simulink model "DatcomNew"  (R2017a)
settings: Solver=VariableStepAuto  StartTime=0.0  StopTime=10.0  RelTol=1e-3
undefined symbols (not defined in the file or in its folder): datcom, Newton, Raphson
libraries: aerolibutil x32, sharedutil x4, aerolibtransform2 x3, aerolibasang x3, aerolibadyn x1
(part 3 of 4)

== system DatcomNew/My Digital DATCOM v1.0.2/Deflection/Aerodynamic Forces and Moments/Force Transformation ==
  Vb : Inport
  Property-In-Stability (PIS) : Inport  Port=2
  Body2Stability : Subsystem
  "Incidence, Sideslip, & Airspeed" : Subsystem
      mask Display:
      | port_label('input',1,'V_b','texmode','on');
      | port_label('output',1,'\alpha','texmode','on');
      | port_label('output',2,'\beta','texmode','on');
      | port_label('output',3,'V','texmode','on');
  Product : Product  Multiplication=Matrix(*)  RndMeth=Zero
  Terminator : Terminator
  Terminator1 : Terminator
  Transpose : Math  Operator=transpose  SaturateOnIntegerOverflow=on
  Property-In-Body (PIB) : Outport
  wires:
  Product/1 -> Property-In-Body (PIB)/1
  Property-In-Stability (PIS)/1 -> Product/2
  "Incidence, Sideslip, & Airspeed"/1(Alpha) -> Body2Stability/1(alpha)
  Body2Stability/1(Ts/b) -> Transpose/1
  Transpose/1 -> Product/1  "Stability2Body"
  Vb/1 -> "Incidence, Sideslip, & Airspeed"/1(Vb)
  "Incidence, Sideslip, & Airspeed"/2(Beta) -> Terminator/1
  "Incidence, Sideslip, & Airspeed"/3(V) -> Terminator1/1

== system DatcomNew/My Digital DATCOM v1.0.2/Deflection/Aerodynamic Forces and Moments/Moment Transformation ==
  Vb : Inport
  Property-In-Stability (PIS) : Inport  Port=2
  Body2Stability : Subsystem
  "Incidence, Sideslip, & Airspeed" : Subsystem
      mask Display:
      | port_label('input',1,'V_b','texmode','on');
      | port_label('output',1,'\alpha','texmode','on');
      | port_label('output',2,'\beta','texmode','on');
      | port_label('output',3,'V','texmode','on');
  Product : Product  Multiplication=Matrix(*)  RndMeth=Zero
  Terminator : Terminator
  Terminator1 : Terminator
  Transpose : Math  Operator=transpose  SaturateOnIntegerOverflow=on
  Property-In-Body (PIB) : Outport
  wires:
  "Incidence, Sideslip, & Airspeed"/3(V) -> Terminator1/1
  "Incidence, Sideslip, & Airspeed"/2(Beta) -> Terminator/1
  Vb/1 -> "Incidence, Sideslip, & Airspeed"/1(Vb)
  Transpose/1 -> Product/1  "Stability2Body"
  Body2Stability/1(Ts/b) -> Transpose/1
  "Incidence, Sideslip, & Airspeed"/1(Alpha) -> Body2Stability/1(alpha)
  Property-In-Stability (PIS)/1 -> Product/2
  Product/1 -> Property-In-Body (PIB)/1

== system DatcomNew/My Digital DATCOM v1.0.2/Deflection/Delta Coefficients/Aileron Deflaction ==
  bus : Inport
  Bus Selector : BusSelector  OutputSignals=idxa,fa,idxm,fm,idxh,fh,idxd_a,fd_a
  Bus Selector1 : BusSelector  OutputSignals=idxa,fa,idxm,fm,idxh,fh,idxd_a,fd_a
  Constant{1,4..6} (4 alike) : Constant  Value=0
  DCl : Interpolation_n-D  NumberOfTableDimensions=4  Table=permute(datcom.dcl_de,[1 2 3 4])  RemoveProtectionIndex=on
      settings: InputPortMap=u0,u1,u2,u3,u4,u5,u6,u7
  DCn : Interpolation_n-D  NumberOfTableDimensions=4  Table=permute(datcom.dcdi_de,[1 2 3 4])  RemoveProtectionIndex=on
      settings: InputPortMap=u0,u1,u2,u3,u4,u5,u6,u7
  Mux1 : Mux  Inputs=6
  delCoeff_a : Outport
  wires:
  Bus Selector/7 -> DCn/7  "<idxd_a>"
  Bus Selector/3 -> DCn/3  "<idxm>"
  Bus Selector1/7 -> DCl/7  "<idxd_a>"
  Bus Selector1/3 -> DCl/3  "<idxm>"
  DCl/1 -> Mux1/4  "Cl_a"
  DCn/1 -> Mux1/6  "Cn_a"
  Constant6/1 -> Mux1/1  "CD_a"
  Constant1/1 -> Mux1/2  "CY_a"
  Constant5/1 -> Mux1/3  "CL_e"
  Constant4/1 -> Mux1/5  "Cm_a"
  bus/1 -> Bus Selector/1, Bus Selector1/1
  Bus Selector1/4 -> DCl/4  "<fm>"
  Bus Selector1/6 -> DCl/6  "<fh>"
  Bus Selector1/8 -> DCl/8  "<fd_a>"
  Bus Selector1/2 -> DCl/2  "<fa>"
  Bus Selector1/5 -> DCl/5  "<idxh>"
  Bus Selector1/1 -> DCl/1  "<idxa>"
  Mux1/1 -> delCoeff_a/1
  Bus Selector/6 -> DCn/6  "<fh>"
  Bus Selector/8 -> DCn/8  "<fd_a>"
  Bus Selector/1 -> DCn/1  "<idxa>"
  Bus Selector/2 -> DCn/2  "<fa>"
  Bus Selector/5 -> DCn/5  "<idxh>"
  Bus Selector/4 -> DCn/4  "<fm>"

== system DatcomNew/My Digital DATCOM v1.0.2/Deflection/Delta Coefficients/Elevator Deflaction ==
  bus : Inport
  Bus Selector : BusSelector  OutputSignals=idxa,fa,idxm,fm,idxh,fh,idxd_e,fd_e
  Bus Selector1 : BusSelector  OutputSignals=idxa,fa,idxm,fm,idxh,fh,idxd_e,fd_e
  Bus Selector2 : BusSelector  OutputSignals=idxa,fa,idxm,fm,idxh,fh,idxd_e,fd_e
  Constant1 : Constant  Value=0
  Constant2 : Constant  Value=0
  Constant3 : Constant  Value=0
  DCDI : Interpolation_n-D  NumberOfTableDimensions=4  Table=permute(datcom.dcdi_de,[1 2 3 4])  RemoveProtectionIndex=on
      settings: InputPortMap=u0,u1,u2,u3,u4,u5,u6,u7
  DCL : Interpolation_n-D  NumberOfTableDimensions=4  Table=permute(datcom.dcl_de,[1 2 3 4])  RemoveProtectionIndex=on
      settings: InputPortMap=u0,u1,u2,u3,u4,u5,u6,u7
  DCm : Interpolation_n-D  NumberOfTableDimensions=4  Table=permute(datcom.dcm_de,[1 2 3 4])  RemoveProtectionIndex=on
      settings: InputPortMap=u0,u1,u2,u3,u4,u5,u6,u7
  Mux1 : Mux  Inputs=6
  delCoeff_e : Outport
  wires:
  Bus Selector2/3 -> DCm/3  "<idxm>"
  Bus Selector2/7 -> DCm/7  "<idxd_e>"
  Bus Selector1/7 -> DCL/7  "<idxd_e>"
  Bus Selector1/3 -> DCL/3  "<idxm>"
  Bus Selector/3 -> DCDI/3  "<idxm>"
  Bus Selector/7 -> DCDI/7  "<idxd_e>"
  Constant2/1 -> Mux1/4  "Cl_e"
  Constant3/1 -> Mux1/6  "Cn_e"
  DCDI/1 -> Mux1/1  "CD_e"
  Constant1/1 -> Mux1/2  "CY_e"
  DCL/1 -> Mux1/3  "CL_e"
  DCm/1 -> Mux1/5  "Cm_e"
  Bus Selector/4 -> DCDI/4  "<fm>"
  Bus Selector/5 -> DCDI/5  "<idxh>"
  Bus Selector/2 -> DCDI/2  "<fa>"
  Bus Selector/1 -> DCDI/1  "<idxa>"
  Bus Selector/8 -> DCDI/8  "<fd_e>"
  Bus Selector/6 -> DCDI/6  "<fh>"
  Mux1/1 -> delCoeff_e/1
  Bus Selector1/1 -> DCL/1  "<idxa>"
  Bus Selector1/5 -> DCL/5  "<idxh>"
  Bus Selector1/2 -> DCL/2  "<fa>"
  Bus Selector2/1 -> DCm/1  "<idxa>"
  Bus Selector2/8 -> DCm/8  "<fd_e>"
  Bus Selector2/5 -> DCm/5  "<idxh>"
  Bus Selector2/4 -> DCm/4  "<fm>"
  Bus Selector2/2 -> DCm/2  "<fa>"
  Bus Selector2/6 -> DCm/6  "<fh>"
  Bus Selector1/8 -> DCL/8  "<fd_e>"
  Bus Selector1/6 -> DCL/6  "<fh>"
  Bus Selector1/4 -> DCL/4  "<fm>"
  bus/1 -> Bus Selector/1, Bus Selector1/1, Bus Selector2/1

== system DatcomNew/My Digital DATCOM v1.0.2/Deflection/Delta Coefficients/Flap Deflaction ==
  bus : Inport
  Bus Selector : BusSelector  OutputSignals=idxa,fa,idxm,fm,idxh,fh,idxd_f,fd_f
  Bus Selector1 : BusSelector  OutputSignals=idxa,fa,idxm,fm,idxh,fh,idxd_f,fd_f
  Bus Selector4 : BusSelector  OutputSignals=idxa,fa,idxm,fm,idxh,fh,idxd_f,fd_f
  Constant1 : Constant  Value=0
  Constant2 : Constant  Value=0
  Constant3 : Constant  Value=0
  DCDI : Interpolation_n-D  NumberOfTableDimensions=4  Table=permute(datcom.dcdi_df,[1 2 3 4])  RemoveProtectionIndex=on
      settings: InputPortMap=u0,u1,u2,u3,u4,u5,u6,u7
  DCL : Interpolation_n-D  NumberOfTableDimensions=4  Table=permute(datcom.dcl_df,[1 2 3 4])  RemoveProtectionIndex=on
      settings: InputPortMap=u0,u1,u2,u3,u4,u5,u6,u7
  DCm : Interpolation_n-D  NumberOfTableDimensions=4  Table=permute(datcom.dcm_df,[1 2 3 4])  RemoveProtectionIndex=on
      settings: InputPortMap=u0,u1,u2,u3,u4,u5,u6,u7
  Mux1 : Mux  Inputs=6
  delCoeff_f : Outport
  wires:
  Bus Selector4/3 -> DCm/3  "<idxm>"
  Bus Selector4/7 -> DCm/7  "<idxd_f>"
  Bus Selector1/7 -> DCL/7  "<idxd_f>"
  Bus Selector1/3 -> DCL/3  "<idxm>"
  Bus Selector/7 -> DCDI/7  "<idxd_f>"
  Bus Selector/3 -> DCDI/3  "<idxm>"
  Constant2/1 -> Mux1/4  "Cl_f"
  Constant3/1 -> Mux1/6  "Cn_f"
  bus/1 -> Bus Selector1/1, Bus Selector4/1, Bus Selector/1
  Bus Selector1/4 -> DCL/4  "<fm>"
  Bus Selector1/6 -> DCL/6  "<fh>"
  DCDI/1 -> Mux1/1  "CD_f"
  Constant1/1 -> Mux1/2  "CY_f"
  DCL/1 -> Mux1/3  "CL_f"
  Bus Selector1/8 -> DCL/8  "<fd_f>"
  Bus Selector4/6 -> DCm/6  "<fh>"
  Bus Selector4/2 -> DCm/2  "<fa>"
  Bus Selector4/4 -> DCm/4  "<fm>"
  Bus Selector4/5 -> DCm/5  "<idxh>"
  Bus Selector4/8 -> DCm/8  "<fd_f>"
  Bus Selector4/1 -> DCm/1  "<idxa>"
  Bus Selector1/2 -> DCL/2  "<fa>"
  Bus Selector1/5 -> DCL/5  "<idxh>"
  Bus Selector1/1 -> DCL/1  "<idxa>"
  DCm/1 -> Mux1/5  "Cm_f"
  Mux1/1 -> delCoeff_f/1
  Bus Selector/6 -> DCDI/6  "<fh>"
  Bus Selector/8 -> DCDI/8  "<fd_f>"
  Bus Selector/1 -> DCDI/1  "<idxa>"
  Bus Selector/2 -> DCDI/2  "<fa>"
  Bus Selector/5 -> DCDI/5  "<idxh>"
  Bus Selector/4 -> DCDI/4  "<fm>"

== system DatcomNew/My Digital DATCOM v1.0.2/Dynamic Contribution/Aerodynamic Forces and Moments Stability Axis/CG-CP Transformation ==
  Vb : Inport
  Property-In-Stability (PIS) : Inport  Port=2
  Body2Stability : Subsystem
  "Incidence, Sideslip, & Airspeed" : Subsystem
      mask Display:
      | port_label('input',1,'V_b','texmode','on');
      | port_label('output',1,'\alpha','texmode','on');
      | port_label('output',2,'\beta','texmode','on');
      | port_label('output',3,'V','texmode','on');
  Product : Product  Multiplication=Matrix(*)  RndMeth=Zero
  Terminator : Terminator
  Terminator1 : Terminator
  Transpose : Math  Operator=transpose  SaturateOnIntegerOverflow=on
  Property-In-Body (PIB) : Outport
  wires:
  Product/1 -> Property-In-Body (PIB)/1
  Property-In-Stability (PIS)/1 -> Product/2
  "Incidence, Sideslip, & Airspeed"/1(Alpha) -> Body2Stability/1(alpha)
  Body2Stability/1(Ts/b) -> Transpose/1
  Transpose/1 -> Product/1  "Stability2Body"
  Vb/1 -> "Incidence, Sideslip, & Airspeed"/1(Vb)
  "Incidence, Sideslip, & Airspeed"/2(Beta) -> Terminator/1
  "Incidence, Sideslip, & Airspeed"/3(V) -> Terminator1/1

== system DatcomNew/My Digital DATCOM v1.0.2/Dynamic Contribution/Aerodynamic Forces and Moments Stability Axis/Force Transformation ==
  Vb : Inport
  Property-In-Stability (PIS) : Inport  Port=2
  Body2Stability : Subsystem
  "Incidence, Sideslip, & Airspeed" : Subsystem
      mask Display:
      | port_label('input',1,'V_b','texmode','on');
      | port_label('output',1,'\alpha','texmode','on');
      | port_label('output',2,'\beta','texmode','on');
      | port_label('output',3,'V','texmode','on');
  Product : Product  Multiplication=Matrix(*)  RndMeth=Zero
  Terminator : Terminator
  Terminator1 : Terminator
  Transpose : Math  Operator=transpose  SaturateOnIntegerOverflow=on
  Property-In-Body (PIB) : Outport
  wires:
  Product/1 -> Property-In-Body (PIB)/1
  Property-In-Stability (PIS)/1 -> Product/2
  "Incidence, Sideslip, & Airspeed"/1(Alpha) -> Body2Stability/1(alpha)
  Body2Stability/1(Ts/b) -> Transpose/1
  Transpose/1 -> Product/1  "Stability2Body"
  Vb/1 -> "Incidence, Sideslip, & Airspeed"/1(Vb)
  "Incidence, Sideslip, & Airspeed"/2(Beta) -> Terminator/1
  "Incidence, Sideslip, & Airspeed"/3(V) -> Terminator1/1

== system DatcomNew/My Digital DATCOM v1.0.2/Dynamic Contribution/Aerodynamic Forces and Moments Stability Axis/Moment Transformation ==
  Vb : Inport
  Property-In-Stability (PIS) : Inport  Port=2
  Body2Stability : Subsystem
  "Incidence, Sideslip, & Airspeed" : Subsystem
      mask Display:
      | port_label('input',1,'V_b','texmode','on');
      | port_label('output',1,'\alpha','texmode','on');
      | port_label('output',2,'\beta','texmode','on');
      | port_label('output',3,'V','texmode','on');
  Product : Product  Multiplication=Matrix(*)  RndMeth=Zero
  Terminator : Terminator
  Terminator1 : Terminator
  Transpose : Math  Operator=transpose  SaturateOnIntegerOverflow=on
  Property-In-Body (PIB) : Outport
  wires:
  "Incidence, Sideslip, & Airspeed"/3(V) -> Terminator1/1
  "Incidence, Sideslip, & Airspeed"/2(Beta) -> Terminator/1
  Vb/1 -> "Incidence, Sideslip, & Airspeed"/1(Vb)
  Transpose/1 -> Product/1  "Stability2Body"
  Body2Stability/1(Ts/b) -> Transpose/1
  "Incidence, Sideslip, & Airspeed"/1(Alpha) -> Body2Stability/1(alpha)
  Property-In-Stability (PIS)/1 -> Product/2
  Product/1 -> Property-In-Body (PIB)/1

== system DatcomNew/My Digital DATCOM v1.0.2/Static Contribution/Aerodynamic Forces and Moments/CG-CP Transformation ==
  Vb : Inport
  Property-In-Stability (PIS) : Inport  Port=2
  Body2Stability : Subsystem
  "Incidence, Sideslip, & Airspeed" : Subsystem
      mask Display:
      | port_label('input',1,'V_b','texmode','on');
      | port_label('output',1,'\alpha','texmode','on');
      | port_label('output',2,'\beta','texmode','on');
      | port_label('output',3,'V','texmode','on');
  Product : Product  Multiplication=Matrix(*)  RndMeth=Zero
  Terminator : Terminator
  Terminator1 : Terminator
  Transpose : Math  Operator=transpose  SaturateOnIntegerOverflow=on
  Property-In-Body (PIB) : Outport
  wires:
  Product/1 -> Property-In-Body (PIB)/1
  Property-In-Stability (PIS)/1 -> Product/2
  "Incidence, Sideslip, & Airspeed"/1(Alpha) -> Body2Stability/1(alpha)
  Body2Stability/1(Ts/b) -> Transpose/1
  Transpose/1 -> Product/1  "Stability2Body"
  Vb/1 -> "Incidence, Sideslip, & Airspeed"/1(Vb)
  "Incidence, Sideslip, & Airspeed"/2(Beta) -> Terminator/1
  "Incidence, Sideslip, & Airspeed"/3(V) -> Terminator1/1

== system DatcomNew/My Digital DATCOM v1.0.2/Static Contribution/Aerodynamic Forces and Moments/Force Transformation ==
  Vb : Inport
  Property-In-Stability (PIS) : Inport  Port=2
  Body2Stability : Subsystem
  "Incidence, Sideslip, & Airspeed" : Subsystem
      mask Display:
      | port_label('input',1,'V_b','texmode','on');
      | port_label('output',1,'\alpha','texmode','on');
      | port_label('output',2,'\beta','texmode','on');
      | port_label('output',3,'V','texmode','on');
  Product : Product  Multiplication=Matrix(*)  RndMeth=Zero
  Terminator : Terminator
  Terminator1 : Terminator
  Transpose : Math  Operator=transpose  SaturateOnIntegerOverflow=on
  Property-In-Body (PIB) : Outport
  wires:
  Product/1 -> Property-In-Body (PIB)/1
  Property-In-Stability (PIS)/1 -> Product/2
  "Incidence, Sideslip, & Airspeed"/1(Alpha) -> Body2Stability/1(alpha)
  Body2Stability/1(Ts/b) -> Transpose/1
  Transpose/1 -> Product/1  "Stability2Body"
  Vb/1 -> "Incidence, Sideslip, & Airspeed"/1(Vb)
  "Incidence, Sideslip, & Airspeed"/2(Beta) -> Terminator/1
  "Incidence, Sideslip, & Airspeed"/3(V) -> Terminator1/1

== system DatcomNew/My Digital DATCOM v1.0.2/Static Contribution/Aerodynamic Forces and Moments/Moment Transformation ==
  Vb : Inport
  Property-In-Stability (PIS) : Inport  Port=2
  Body2Stability : Subsystem
  "Incidence, Sideslip, & Airspeed" : Subsystem
      mask Display:
      | port_label('input',1,'V_b','texmode','on');
      | port_label('output',1,'\alpha','texmode','on');
      | port_label('output',2,'\beta','texmode','on');
      | port_label('output',3,'V','texmode','on');
  Product : Product  Multiplication=Matrix(*)  RndMeth=Zero
  Terminator : Terminator
  Terminator1 : Terminator
  Transpose : Math  Operator=transpose  SaturateOnIntegerOverflow=on
  Property-In-Body (PIB) : Outport
  wires:
  "Incidence, Sideslip, & Airspeed"/3(V) -> Terminator1/1
  "Incidence, Sideslip, & Airspeed"/2(Beta) -> Terminator/1
  Vb/1 -> "Incidence, Sideslip, & Airspeed"/1(Vb)
  Transpose/1 -> Product/1  "Stability2Body"
  Body2Stability/1(Ts/b) -> Transpose/1
  "Incidence, Sideslip, & Airspeed"/1(Alpha) -> Body2Stability/1(alpha)
  Property-In-Stability (PIS)/1 -> Product/2
  Product/1 -> Property-In-Body (PIB)/1

== system DatcomNew/My Digital DATCOM v1.0.3/Deflection/Aerodynamic Forces and Moments/CG-CP Transformation ==
  Vb : Inport
  Property-In-Stability (PIS) : Inport  Port=2
  Body2Stability : Subsystem
  "Incidence, Sideslip, & Airspeed" : Subsystem
      mask Display:
      | port_label('input',1,'V_b','texmode','on');
      | port_label('output',1,'\alpha','texmode','on');
      | port_label('output',2,'\beta','texmode','on');
      | port_label('output',3,'V','texmode','on');
  Product : Product  Multiplication=Matrix(*)  RndMeth=Zero
  Terminator : Terminator
  Terminator1 : Terminator
  Transpose : Math  Operator=transpose  SaturateOnIntegerOverflow=on
  Property-In-Body (PIB) : Outport
  wires:
  Product/1 -> Property-In-Body (PIB)/1
  Property-In-Stability (PIS)/1 -> Product/2
  "Incidence, Sideslip, & Airspeed"/1(Alpha) -> Body2Stability/1(alpha)
  Body2Stability/1(Ts/b) -> Transpose/1
  Transpose/1 -> Product/1  "Stability2Body"
  Vb/1 -> "Incidence, Sideslip, & Airspeed"/1(Vb)
  "Incidence, Sideslip, & Airspeed"/2(Beta) -> Terminator/1
  "Incidence, Sideslip, & Airspeed"/3(V) -> Terminator1/1

== system DatcomNew/My Digital DATCOM v1.0.3/Deflection/Aerodynamic Forces and Moments/Force Transformation ==
  Vb : Inport
  Property-In-Stability (PIS) : Inport  Port=2
  Body2Stability : Subsystem
  "Incidence, Sideslip, & Airspeed" : Subsystem
      mask Display:
      | port_label('input',1,'V_b','texmode','on');
      | port_label('output',1,'\alpha','texmode','on');
      | port_label('output',2,'\beta','texmode','on');
      | port_label('output',3,'V','texmode','on');
  Product : Product  Multiplication=Matrix(*)  RndMeth=Zero
  Terminator : Terminator
  Terminator1 : Terminator
  Transpose : Math  Operator=transpose  SaturateOnIntegerOverflow=on
  Property-In-Body (PIB) : Outport
  wires:
  Product/1 -> Property-In-Body (PIB)/1
  Property-In-Stability (PIS)/1 -> Product/2
  "Incidence, Sideslip, & Airspeed"/1(Alpha) -> Body2Stability/1(alpha)
  Body2Stability/1(Ts/b) -> Transpose/1
  Transpose/1 -> Product/1  "Stability2Body"
  Vb/1 -> "Incidence, Sideslip, & Airspeed"/1(Vb)
  "Incidence, Sideslip, & Airspeed"/2(Beta) -> Terminator/1
  "Incidence, Sideslip, & Airspeed"/3(V) -> Terminator1/1

== system DatcomNew/My Digital DATCOM v1.0.3/Deflection/Aerodynamic Forces and Moments/Moment Transformation ==
  Vb : Inport
  Property-In-Stability (PIS) : Inport  Port=2
  Body2Stability : Subsystem
  "Incidence, Sideslip, & Airspeed" : Subsystem
      mask Display:
      | port_label('input',1,'V_b','texmode','on');
      | port_label('output',1,'\alpha','texmode','on');
      | port_label('output',2,'\beta','texmode','on');
      | port_label('output',3,'V','texmode','on');
  Product : Product  Multiplication=Matrix(*)  RndMeth=Zero
  Terminator : Terminator
  Terminator1 : Terminator
  Transpose : Math  Operator=transpose  SaturateOnIntegerOverflow=on
  Property-In-Body (PIB) : Outport
  wires:
  "Incidence, Sideslip, & Airspeed"/3(V) -> Terminator1/1
  "Incidence, Sideslip, & Airspeed"/2(Beta) -> Terminator/1
  Vb/1 -> "Incidence, Sideslip, & Airspeed"/1(Vb)
  Transpose/1 -> Product/1  "Stability2Body"
  Body2Stability/1(Ts/b) -> Transpose/1
  "Incidence, Sideslip, & Airspeed"/1(Alpha) -> Body2Stability/1(alpha)
  Property-In-Stability (PIS)/1 -> Product/2
  Product/1 -> Property-In-Body (PIB)/1

== system DatcomNew/My Digital DATCOM v1.0.3/Deflection/Delta Coefficients/Aileron Deflaction ==
  bus : Inport
  Bus Selector : BusSelector  OutputSignals=idxa,fa,idxm,fm,idxh,fh,idxd_a,fd_a
  Bus Selector1 : BusSelector  OutputSignals=idxa,fa,idxm,fm,idxh,fh,idxd_a,fd_a
  Constant{1,4..6} (4 alike) : Constant  Value=0
  DCl : Interpolation_n-D  NumberOfTableDimensions=4  Table=permute(datcom.dcl_de,[1 2 3 4])  RemoveProtectionIndex=on
      settings: InputPortMap=u0,u1,u2,u3,u4,u5,u6,u7
  DCn : Interpolation_n-D  NumberOfTableDimensions=4  Table=permute(datcom.dcdi_de,[1 2 3 4])  RemoveProtectionIndex=on
      settings: InputPortMap=u0,u1,u2,u3,u4,u5,u6,u7
  Mux1 : Mux  Inputs=6
  delCoeff_a : Outport
  wires:
  Bus Selector/7 -> DCn/7  "<idxd_a>"
  Bus Selector/3 -> DCn/3  "<idxm>"
  Bus Selector1/7 -> DCl/7  "<idxd_a>"
  Bus Selector1/3 -> DCl/3  "<idxm>"
  DCl/1 -> Mux1/4  "Cl_a"
  DCn/1 -> Mux1/6  "Cn_a"
  Constant6/1 -> Mux1/1  "CD_a"
  Constant1/1 -> Mux1/2  "CY_a"
  Constant5/1 -> Mux1/3  "CL_e"
  Constant4/1 -> Mux1/5  "Cm_a"
  bus/1 -> Bus Selector/1, Bus Selector1/1
  Bus Selector1/4 -> DCl/4  "<fm>"
  Bus Selector1/6 -> DCl/6  "<fh>"
  Bus Selector1/8 -> DCl/8  "<fd_a>"
  Bus Selector1/2 -> DCl/2  "<fa>"
  Bus Selector1/5 -> DCl/5  "<idxh>"
  Bus Selector1/1 -> DCl/1  "<idxa>"
  Mux1/1 -> delCoeff_a/1
  Bus Selector/6 -> DCn/6  "<fh>"
  Bus Selector/8 -> DCn/8  "<fd_a>"
  Bus Selector/1 -> DCn/1  "<idxa>"
  Bus Selector/2 -> DCn/2  "<fa>"
  Bus Selector/5 -> DCn/5  "<idxh>"
  Bus Selector/4 -> DCn/4  "<fm>"

== system DatcomNew/My Digital DATCOM v1.0.3/Deflection/Delta Coefficients/Elevator Deflaction ==
  bus : Inport
  Bus Selector : BusSelector  OutputSignals=idxa,fa,idxm,fm,idxh,fh,idxd_e,fd_e
  Bus Selector1 : BusSelector  OutputSignals=idxa,fa,idxm,fm,idxh,fh,idxd_e,fd_e
  Bus Selector2 : BusSelector  OutputSignals=idxa,fa,idxm,fm,idxh,fh,idxd_e,fd_e
  Constant1 : Constant  Value=0
  Constant2 : Constant  Value=0
  Constant3 : Constant  Value=0
  DCDI : Interpolation_n-D  NumberOfTableDimensions=4  Table=permute(datcom.dcdi_de,[1 2 3 4])  RemoveProtectionIndex=on
      settings: InputPortMap=u0,u1,u2,u3,u4,u5,u6,u7
  DCL : Interpolation_n-D  NumberOfTableDimensions=4  Table=permute(datcom.dcl_de,[1 2 3 4])  RemoveProtectionIndex=on
      settings: InputPortMap=u0,u1,u2,u3,u4,u5,u6,u7
  DCm : Interpolation_n-D  NumberOfTableDimensions=4  Table=permute(datcom.dcm_de,[1 2 3 4])  RemoveProtectionIndex=on
      settings: InputPortMap=u0,u1,u2,u3,u4,u5,u6,u7
  Mux1 : Mux  Inputs=6
  delCoeff_e : Outport
  wires:
  Bus Selector2/3 -> DCm/3  "<idxm>"
  Bus Selector2/7 -> DCm/7  "<idxd_e>"
  Bus Selector1/7 -> DCL/7  "<idxd_e>"
  Bus Selector1/3 -> DCL/3  "<idxm>"
  Bus Selector/3 -> DCDI/3  "<idxm>"
  Bus Selector/7 -> DCDI/7  "<idxd_e>"
  Constant2/1 -> Mux1/4  "Cl_e"
  Constant3/1 -> Mux1/6  "Cn_e"
  DCDI/1 -> Mux1/1  "CD_e"
  Constant1/1 -> Mux1/2  "CY_e"
  DCL/1 -> Mux1/3  "CL_e"
  DCm/1 -> Mux1/5  "Cm_e"
  Bus Selector/4 -> DCDI/4  "<fm>"
  Bus Selector/5 -> DCDI/5  "<idxh>"
  Bus Selector/2 -> DCDI/2  "<fa>"
  Bus Selector/1 -> DCDI/1  "<idxa>"
  Bus Selector/8 -> DCDI/8  "<fd_e>"
  Bus Selector/6 -> DCDI/6  "<fh>"
  Mux1/1 -> delCoeff_e/1
  Bus Selector1/1 -> DCL/1  "<idxa>"
  Bus Selector1/5 -> DCL/5  "<idxh>"
  Bus Selector1/2 -> DCL/2  "<fa>"
  Bus Selector2/1 -> DCm/1  "<idxa>"
  Bus Selector2/8 -> DCm/8  "<fd_e>"
  Bus Selector2/5 -> DCm/5  "<idxh>"
  Bus Selector2/4 -> DCm/4  "<fm>"
  Bus Selector2/2 -> DCm/2  "<fa>"
  Bus Selector2/6 -> DCm/6  "<fh>"
  Bus Selector1/8 -> DCL/8  "<fd_e>"
  Bus Selector1/6 -> DCL/6  "<fh>"
  Bus Selector1/4 -> DCL/4  "<fm>"
  bus/1 -> Bus Selector/1, Bus Selector1/1, Bus Selector2/1

== system DatcomNew/My Digital DATCOM v1.0.3/Deflection/Delta Coefficients/Flap Deflaction ==
  bus : Inport
  Bus Selector : BusSelector  OutputSignals=idxa,fa,idxm,fm,idxh,fh,idxd_f,fd_f
  Bus Selector1 : BusSelector  OutputSignals=idxa,fa,idxm,fm,idxh,fh,idxd_f,fd_f
  Bus Selector4 : BusSelector  OutputSignals=idxa,fa,idxm,fm,idxh,fh,idxd_f,fd_f
  Constant1 : Constant  Value=0
  Constant2 : Constant  Value=0
  Constant3 : Constant  Value=0
  DCDI : Interpolation_n-D  NumberOfTableDimensions=4  Table=permute(datcom.dcdi_df,[1 2 3 4])  RemoveProtectionIndex=on
      settings: InputPortMap=u0,u1,u2,u3,u4,u5,u6,u7
  DCL : Interpolation_n-D  NumberOfTableDimensions=4  Table=permute(datcom.dcl_df,[1 2 3 4])  RemoveProtectionIndex=on
      settings: InputPortMap=u0,u1,u2,u3,u4,u5,u6,u7
  DCm : Interpolation_n-D  NumberOfTableDimensions=4  Table=permute(datcom.dcm_df,[1 2 3 4])  RemoveProtectionIndex=on
      settings: InputPortMap=u0,u1,u2,u3,u4,u5,u6,u7
  Mux1 : Mux  Inputs=6
  delCoeff_f : Outport
  wires:
  Bus Selector4/3 -> DCm/3  "<idxm>"
  Bus Selector4/7 -> DCm/7  "<idxd_f>"
  Bus Selector1/7 -> DCL/7  "<idxd_f>"
  Bus Selector1/3 -> DCL/3  "<idxm>"
  Bus Selector/7 -> DCDI/7  "<idxd_f>"
  Bus Selector/3 -> DCDI/3  "<idxm>"
  Constant2/1 -> Mux1/4  "Cl_f"
  Constant3/1 -> Mux1/6  "Cn_f"
  bus/1 -> Bus Selector1/1, Bus Selector4/1, Bus Selector/1
  Bus Selector1/4 -> DCL/4  "<fm>"
  Bus Selector1/6 -> DCL/6  "<fh>"
  DCDI/1 -> Mux1/1  "CD_f"
  Constant1/1 -> Mux1/2  "CY_f"
  DCL/1 -> Mux1/3  "CL_f"
  Bus Selector1/8 -> DCL/8  "<fd_f>"
  Bus Selector4/6 -> DCm/6  "<fh>"
  Bus Selector4/2 -> DCm/2  "<fa>"
  Bus Selector4/4 -> DCm/4  "<fm>"
  Bus Selector4/5 -> DCm/5  "<idxh>"
  Bus Selector4/8 -> DCm/8  "<fd_f>"
  Bus Selector4/1 -> DCm/1  "<idxa>"
  Bus Selector1/2 -> DCL/2  "<fa>"
  Bus Selector1/5 -> DCL/5  "<idxh>"
  Bus Selector1/1 -> DCL/1  "<idxa>"
  DCm/1 -> Mux1/5  "Cm_f"
  Mux1/1 -> delCoeff_f/1
  Bus Selector/6 -> DCDI/6  "<fh>"
  Bus Selector/8 -> DCDI/8  "<fd_f>"
  Bus Selector/1 -> DCDI/1  "<idxa>"
  Bus Selector/2 -> DCDI/2  "<fa>"
  Bus Selector/5 -> DCDI/5  "<idxh>"
  Bus Selector/4 -> DCDI/4  "<fm>"

== system DatcomNew/My Digital DATCOM v1.0.3/Dynamic Contribution/Aerodynamic Forces and Moments Stability Axis/CG-CP Transformation ==
  Vb : Inport
  Property-In-Stability (PIS) : Inport  Port=2
  Body2Stability : Subsystem
  "Incidence, Sideslip, & Airspeed" : Subsystem
      mask Display:
      | port_label('input',1,'V_b','texmode','on');
      | port_label('output',1,'\alpha','texmode','on');
      | port_label('output',2,'\beta','texmode','on');
      | port_label('output',3,'V','texmode','on');
  Product : Product  Multiplication=Matrix(*)  RndMeth=Zero
  Terminator : Terminator
  Terminator1 : Terminator
  Transpose : Math  Operator=transpose  SaturateOnIntegerOverflow=on
  Property-In-Body (PIB) : Outport
  wires:
  Product/1 -> Property-In-Body (PIB)/1
  Property-In-Stability (PIS)/1 -> Product/2
  "Incidence, Sideslip, & Airspeed"/1(Alpha) -> Body2Stability/1(alpha)
  Body2Stability/1(Ts/b) -> Transpose/1
  Transpose/1 -> Product/1  "Stability2Body"
  Vb/1 -> "Incidence, Sideslip, & Airspeed"/1(Vb)
  "Incidence, Sideslip, & Airspeed"/2(Beta) -> Terminator/1
  "Incidence, Sideslip, & Airspeed"/3(V) -> Terminator1/1

== system DatcomNew/My Digital DATCOM v1.0.3/Dynamic Contribution/Aerodynamic Forces and Moments Stability Axis/Force Transformation ==
  Vb : Inport
  Property-In-Stability (PIS) : Inport  Port=2
  Body2Stability : Subsystem
  "Incidence, Sideslip, & Airspeed" : Subsystem
      mask Display:
      | port_label('input',1,'V_b','texmode','on');
      | port_label('output',1,'\alpha','texmode','on');
      | port_label('output',2,'\beta','texmode','on');
      | port_label('output',3,'V','texmode','on');
  Product : Product  Multiplication=Matrix(*)  RndMeth=Zero
  Terminator : Terminator
  Terminator1 : Terminator
  Transpose : Math  Operator=transpose  SaturateOnIntegerOverflow=on
  Property-In-Body (PIB) : Outport
  wires:
  Product/1 -> Property-In-Body (PIB)/1
  Property-In-Stability (PIS)/1 -> Product/2
  "Incidence, Sideslip, & Airspeed"/1(Alpha) -> Body2Stability/1(alpha)
  Body2Stability/1(Ts/b) -> Transpose/1
  Transpose/1 -> Product/1  "Stability2Body"
  Vb/1 -> "Incidence, Sideslip, & Airspeed"/1(Vb)
  "Incidence, Sideslip, & Airspeed"/2(Beta) -> Terminator/1
  "Incidence, Sideslip, & Airspeed"/3(V) -> Terminator1/1

== system DatcomNew/My Digital DATCOM v1.0.3/Dynamic Contribution/Aerodynamic Forces and Moments Stability Axis/Moment Transformation ==
  Vb : Inport
  Property-In-Stability (PIS) : Inport  Port=2
  Body2Stability : Subsystem
  "Incidence, Sideslip, & Airspeed" : Subsystem
      mask Display:
      | port_label('input',1,'V_b','texmode','on');
      | port_label('output',1,'\alpha','texmode','on');
      | port_label('output',2,'\beta','texmode','on');
      | port_label('output',3,'V','texmode','on');
  Product : Product  Multiplication=Matrix(*)  RndMeth=Zero
  Terminator : Terminator
  Terminator1 : Terminator
  Transpose : Math  Operator=transpose  SaturateOnIntegerOverflow=on
  Property-In-Body (PIB) : Outport
  wires:
  "Incidence, Sideslip, & Airspeed"/3(V) -> Terminator1/1
  "Incidence, Sideslip, & Airspeed"/2(Beta) -> Terminator/1
  Vb/1 -> "Incidence, Sideslip, & Airspeed"/1(Vb)
  Transpose/1 -> Product/1  "Stability2Body"
  Body2Stability/1(Ts/b) -> Transpose/1
  "Incidence, Sideslip, & Airspeed"/1(Alpha) -> Body2Stability/1(alpha)
  Property-In-Stability (PIS)/1 -> Product/2
  Product/1 -> Property-In-Body (PIB)/1

== system DatcomNew/My Digital DATCOM v1.0.3/Static Contribution/Aerodynamic Forces and Moments/CG-CP Transformation ==
  Vb : Inport
  Property-In-Stability (PIS) : Inport  Port=2
  Body2Stability : Subsystem
  "Incidence, Sideslip, & Airspeed" : Subsystem
      mask Display:
      | port_label('input',1,'V_b','texmode','on');
      | port_label('output',1,'\alpha','texmode','on');
      | port_label('output',2,'\beta','texmode','on');
      | port_label('output',3,'V','texmode','on');
  Product : Product  Multiplication=Matrix(*)  RndMeth=Zero
  Terminator : Terminator
  Terminator1 : Terminator
  Transpose : Math  Operator=transpose  SaturateOnIntegerOverflow=on
  Property-In-Body (PIB) : Outport
  wires:
  Product/1 -> Property-In-Body (PIB)/1
  Property-In-Stability (PIS)/1 -> Product/2
  "Incidence, Sideslip, & Airspeed"/1(Alpha) -> Body2Stability/1(alpha)
  Body2Stability/1(Ts/b) -> Transpose/1
  Transpose/1 -> Product/1  "Stability2Body"
  Vb/1 -> "Incidence, Sideslip, & Airspeed"/1(Vb)
  "Incidence, Sideslip, & Airspeed"/2(Beta) -> Terminator/1
  "Incidence, Sideslip, & Airspeed"/3(V) -> Terminator1/1

== system DatcomNew/My Digital DATCOM v1.0.3/Static Contribution/Aerodynamic Forces and Moments/Force Transformation ==
  Vb : Inport
  Property-In-Stability (PIS) : Inport  Port=2
  Body2Stability : Subsystem
  "Incidence, Sideslip, & Airspeed" : Subsystem
      mask Display:
      | port_label('input',1,'V_b','texmode','on');
      | port_label('output',1,'\alpha','texmode','on');
      | port_label('output',2,'\beta','texmode','on');
      | port_label('output',3,'V','texmode','on');
  Product : Product  Multiplication=Matrix(*)  RndMeth=Zero
  Terminator : Terminator
  Terminator1 : Terminator
  Transpose : Math  Operator=transpose  SaturateOnIntegerOverflow=on
  Property-In-Body (PIB) : Outport
  wires:
  Product/1 -> Property-In-Body (PIB)/1
  Property-In-Stability (PIS)/1 -> Product/2
  "Incidence, Sideslip, & Airspeed"/1(Alpha) -> Body2Stability/1(alpha)
  Body2Stability/1(Ts/b) -> Transpose/1
  Transpose/1 -> Product/1  "Stability2Body"
  Vb/1 -> "Incidence, Sideslip, & Airspeed"/1(Vb)
  "Incidence, Sideslip, & Airspeed"/2(Beta) -> Terminator/1
  "Incidence, Sideslip, & Airspeed"/3(V) -> Terminator1/1

== system DatcomNew/My Digital DATCOM v1.0.3/Static Contribution/Aerodynamic Forces and Moments/Moment Transformation ==
  Vb : Inport
  Property-In-Stability (PIS) : Inport  Port=2
  Body2Stability : Subsystem
  "Incidence, Sideslip, & Airspeed" : Subsystem
      mask Display:
      | port_label('input',1,'V_b','texmode','on');
      | port_label('output',1,'\alpha','texmode','on');
      | port_label('output',2,'\beta','texmode','on');
      | port_label('output',3,'V','texmode','on');
  Product : Product  Multiplication=Matrix(*)  RndMeth=Zero
  Terminator : Terminator
  Terminator1 : Terminator
  Transpose : Math  Operator=transpose  SaturateOnIntegerOverflow=on
  Property-In-Body (PIB) : Outport
  wires:
  "Incidence, Sideslip, & Airspeed"/3(V) -> Terminator1/1
  "Incidence, Sideslip, & Airspeed"/2(Beta) -> Terminator/1
  Vb/1 -> "Incidence, Sideslip, & Airspeed"/1(Vb)
  Transpose/1 -> Product/1  "Stability2Body"
  Body2Stability/1(Ts/b) -> Transpose/1
  "Incidence, Sideslip, & Airspeed"/1(Alpha) -> Body2Stability/1(alpha)
  Property-In-Stability (PIS)/1 -> Product/2
  Product/1 -> Property-In-Body (PIB)/1

== system DatcomNew/My Digital DATCOM v1.0.1/Deflection/Aerodynamic Forces and Moments/CG-CP Transformation/Body2Stability ==
  alpha : Inport
  Constant{,1,3..4} (4 alike) : Constant  Value=0
  Constant2 : Constant
  Create 3x3 Matrix : aerolibutil/Create 3x3 Matrix
      settings: SourceProductName=Aerospace Blockset  SourceProductBaseCode=AE
  Trigonometric Function2 : Trigonometry  Operator=sincos
  Unary Minus : UnaryMinus
  Ts/b : Outport
  wires:
  Create 3x3 Matrix/1 -> Ts/b/1
  Constant/1 -> Create 3x3 Matrix/2
  Constant1/1 -> Create 3x3 Matrix/4
  Constant2/1 -> Create 3x3 Matrix/5
  Constant3/1 -> Create 3x3 Matrix/6
  Trigonometric Function2/1 -> Create 3x3 Matrix/3, Unary Minus/1
  Unary Minus/1 -> Create 3x3 Matrix/7
  Constant4/1 -> Create 3x3 Matrix/8
  Trigonometric Function2/2 -> Create 3x3 Matrix/1, Create 3x3 Matrix/9
  alpha/1 -> Trigonometric Function2/1

== system DatcomNew/My Digital DATCOM v1.0.1/Deflection/Aerodynamic Forces and Moments/CG-CP Transformation/Incidence, Sideslip, & Airspeed ==
  Vb : Inport  Unit=m/s
  Airspeed : Sqrt  AlgorithmType=Newton-Raphson  SaturateOnIntegerOverflow=on
  Dot Product : DotProduct  InputSameDT=on  OutDataTypeStr=Inherit: Inherit via internal rule
  Incidence : Trigonometry  Operator=atan2
  Product : Product  Inputs=*/  SaturateOnIntegerOverflow=on  OutDataTypeStr=Inherit: Same as first input
  Selector : Selector  InputPortWidth=3  IndexOptions=Index vector (dialog)  Indices=[2]  OutputSizes=1
  Selector1 : Selector  InputPortWidth=3  IndexOptions=Index vector (dialog)  Indices=[3]  OutputSizes=1
  Selector2 : Selector  InputPortWidth=3  IndexOptions=Index vector (dialog)  Indices=[1]  OutputSizes=1
  Sideslip : Trigonometry  Operator=asin
  Alpha : Outport  Unit=rad  InitialOutput=0
  Beta : Outport  Port=2  Unit=rad  InitialOutput=0
  V : Outport  Port=3  Unit=m/s  InitialOutput=0
  wires:
  Product/1 -> Sideslip/1
  Selector1/1 -> Incidence/1
  Selector2/1 -> Incidence/2
  Dot Product/1 -> Airspeed/1
  Airspeed/1 -> Product/2, V/1
  Incidence/1 -> Alpha/1
  Vb/1 -> Selector1/1, Selector2/1, Selector/1, Dot Product/1, Dot Product/2
  Sideslip/1 -> Beta/1
  Selector/1 -> Product/1

== system DatcomNew/My Digital DATCOM v1.0.1/Deflection/Aerodynamic Forces and Moments/Force Transformation/Body2Stability ==
  alpha : Inport
  Constant{,1,3..4} (4 alike) : Constant  Value=0
  Constant2 : Constant
  Create 3x3 Matrix : aerolibutil/Create 3x3 Matrix
      settings: SourceProductName=Aerospace Blockset  SourceProductBaseCode=AE
  Trigonometric Function2 : Trigonometry  Operator=sincos
  Unary Minus : UnaryMinus
  Ts/b : Outport
  wires:
  Create 3x3 Matrix/1 -> Ts/b/1
  Constant/1 -> Create 3x3 Matrix/2
  Constant1/1 -> Create 3x3 Matrix/4
  Constant2/1 -> Create 3x3 Matrix/5
  Constant3/1 -> Create 3x3 Matrix/6
  Trigonometric Function2/1 -> Create 3x3 Matrix/3, Unary Minus/1
  Unary Minus/1 -> Create 3x3 Matrix/7
  Constant4/1 -> Create 3x3 Matrix/8
  Trigonometric Function2/2 -> Create 3x3 Matrix/1, Create 3x3 Matrix/9
  alpha/1 -> Trigonometric Function2/1

== system DatcomNew/My Digital DATCOM v1.0.1/Deflection/Aerodynamic Forces and Moments/Force Transformation/Incidence, Sideslip, & Airspeed ==
  Vb : Inport  Unit=m/s
  Airspeed : Sqrt  AlgorithmType=Newton-Raphson  SaturateOnIntegerOverflow=on
  Dot Product : DotProduct  InputSameDT=on  OutDataTypeStr=Inherit: Inherit via internal rule
  Incidence : Trigonometry  Operator=atan2
  Product : Product  Inputs=*/  SaturateOnIntegerOverflow=on  OutDataTypeStr=Inherit: Same as first input
  Selector : Selector  InputPortWidth=3  IndexOptions=Index vector (dialog)  Indices=[2]  OutputSizes=1
  Selector1 : Selector  InputPortWidth=3  IndexOptions=Index vector (dialog)  Indices=[3]  OutputSizes=1
  Selector2 : Selector  InputPortWidth=3  IndexOptions=Index vector (dialog)  Indices=[1]  OutputSizes=1
  Sideslip : Trigonometry  Operator=asin
  Alpha : Outport  Unit=rad  InitialOutput=0
  Beta : Outport  Port=2  Unit=rad  InitialOutput=0
  V : Outport  Port=3  Unit=m/s  InitialOutput=0
  wires:
  Product/1 -> Sideslip/1
  Selector1/1 -> Incidence/1
  Selector2/1 -> Incidence/2
  Dot Product/1 -> Airspeed/1
  Airspeed/1 -> Product/2, V/1
  Incidence/1 -> Alpha/1
  Vb/1 -> Selector1/1, Selector2/1, Selector/1, Dot Product/1, Dot Product/2
  Sideslip/1 -> Beta/1
  Selector/1 -> Product/1

== system DatcomNew/My Digital DATCOM v1.0.1/Deflection/Aerodynamic Forces and Moments/Moment Transformation/Body2Stability ==
  alpha : Inport
  Constant{,1,3..4} (4 alike) : Constant  Value=0
  Constant2 : Constant
  Create 3x3 Matrix : aerolibutil/Create 3x3 Matrix
      settings: SourceProductName=Aerospace Blockset  SourceProductBaseCode=AE
  Trigonometric Function2 : Trigonometry  Operator=sincos
  Unary Minus : UnaryMinus
  Ts/b : Outport
  wires:
  alpha/1 -> Trigonometric Function2/1
  Trigonometric Function2/2 -> Create 3x3 Matrix/9, Create 3x3 Matrix/1
  Constant4/1 -> Create 3x3 Matrix/8
  Unary Minus/1 -> Create 3x3 Matrix/7
  Trigonometric Function2/1 -> Unary Minus/1, Create 3x3 Matrix/3
  Constant3/1 -> Create 3x3 Matrix/6
  Constant2/1 -> Create 3x3 Matrix/5
  Constant1/1 -> Create 3x3 Matrix/4
  Constant/1 -> Create 3x3 Matrix/2
  Create 3x3 Matrix/1 -> Ts/b/1

== system DatcomNew/My Digital DATCOM v1.0.1/Deflection/Aerodynamic Forces and Moments/Moment Transformation/Incidence, Sideslip, & Airspeed ==
  Vb : Inport  Unit=m/s
  Airspeed : Sqrt  AlgorithmType=Newton-Raphson  SaturateOnIntegerOverflow=on
  Dot Product : DotProduct  InputSameDT=on  OutDataTypeStr=Inherit: Inherit via internal rule
  Incidence : Trigonometry  Operator=atan2
  Product : Product  Inputs=*/  SaturateOnIntegerOverflow=on  OutDataTypeStr=Inherit: Same as first input
  Selector : Selector  InputPortWidth=3  IndexOptions=Index vector (dialog)  Indices=[2]  OutputSizes=1
  Selector1 : Selector  InputPortWidth=3  IndexOptions=Index vector (dialog)  Indices=[3]  OutputSizes=1
  Selector2 : Selector  InputPortWidth=3  IndexOptions=Index vector (dialog)  Indices=[1]  OutputSizes=1
  Sideslip : Trigonometry  Operator=asin
  Alpha : Outport  Unit=rad  InitialOutput=0
  Beta : Outport  Port=2  Unit=rad  InitialOutput=0
  V : Outport  Port=3  Unit=m/s  InitialOutput=0
  wires:
  Selector/1 -> Product/1
  Sideslip/1 -> Beta/1
  Vb/1 -> Dot Product/2, Dot Product/1, Selector/1, Selector2/1, Selector1/1
  Incidence/1 -> Alpha/1
  Airspeed/1 -> V/1, Product/2
  Dot Product/1 -> Airspeed/1
  Selector2/1 -> Incidence/2
  Selector1/1 -> Incidence/1
  Product/1 -> Sideslip/1

== system DatcomNew/My Digital DATCOM v1.0.1/Dynamic Contribution/Aerodynamic Forces and Moments Stability Axis/CG-CP Transformation/Body2Stability ==
  alpha : Inport
  Constant{,1,3..4} (4 alike) : Constant  Value=0
  Constant2 : Constant
  Create 3x3 Matrix : aerolibutil/Create 3x3 Matrix
      settings: SourceProductName=Aerospace Blockset  SourceProductBaseCode=AE
  Trigonometric Function2 : Trigonometry  Operator=sincos
  Unary Minus : UnaryMinus
  Ts/b : Outport
  wires:
  Create 3x3 Matrix/1 -> Ts/b/1
  Constant/1 -> Create 3x3 Matrix/2
  Constant1/1 -> Create 3x3 Matrix/4
  Constant2/1 -> Create 3x3 Matrix/5
  Constant3/1 -> Create 3x3 Matrix/6
  Trigonometric Function2/1 -> Create 3x3 Matrix/3, Unary Minus/1
  Unary Minus/1 -> Create 3x3 Matrix/7
  Constant4/1 -> Create 3x3 Matrix/8
  Trigonometric Function2/2 -> Create 3x3 Matrix/1, Create 3x3 Matrix/9
  alpha/1 -> Trigonometric Function2/1

== system DatcomNew/My Digital DATCOM v1.0.1/Dynamic Contribution/Aerodynamic Forces and Moments Stability Axis/CG-CP Transformation/Incidence, Sideslip, & Airspeed ==
  Vb : Inport  Unit=m/s
  Airspeed : Sqrt  AlgorithmType=Newton-Raphson  SaturateOnIntegerOverflow=on
  Dot Product : DotProduct  InputSameDT=on  OutDataTypeStr=Inherit: Inherit via internal rule
  Incidence : Trigonometry  Operator=atan2
  Product : Product  Inputs=*/  SaturateOnIntegerOverflow=on  OutDataTypeStr=Inherit: Same as first input
  Selector : Selector  InputPortWidth=3  IndexOptions=Index vector (dialog)  Indices=[2]  OutputSizes=1
  Selector1 : Selector  InputPortWidth=3  IndexOptions=Index vector (dialog)  Indices=[3]  OutputSizes=1
  Selector2 : Selector  InputPortWidth=3  IndexOptions=Index vector (dialog)  Indices=[1]  OutputSizes=1
  Sideslip : Trigonometry  Operator=asin
  Alpha : Outport  Unit=rad  InitialOutput=0
  Beta : Outport  Port=2  Unit=rad  InitialOutput=0
  V : Outport  Port=3  Unit=m/s  InitialOutput=0
  wires:
  Product/1 -> Sideslip/1
  Selector1/1 -> Incidence/1
  Selector2/1 -> Incidence/2
  Dot Product/1 -> Airspeed/1
  Airspeed/1 -> Product/2, V/1
  Incidence/1 -> Alpha/1
  Vb/1 -> Selector1/1, Selector2/1, Selector/1, Dot Product/1, Dot Product/2
  Sideslip/1 -> Beta/1
  Selector/1 -> Product/1

== system DatcomNew/My Digital DATCOM v1.0.1/Dynamic Contribution/Aerodynamic Forces and Moments Stability Axis/Force Transformation/Body2Stability ==
  alpha : Inport
  Constant{,1,3..4} (4 alike) : Constant  Value=0
  Constant2 : Constant
  Create 3x3 Matrix : aerolibutil/Create 3x3 Matrix
      settings: SourceProductName=Aerospace Blockset  SourceProductBaseCode=AE
  Trigonometric Function2 : Trigonometry  Operator=sincos
  Unary Minus : UnaryMinus
  Ts/b : Outport
  wires:
  Create 3x3 Matrix/1 -> Ts/b/1
  Constant/1 -> Create 3x3 Matrix/2
  Constant1/1 -> Create 3x3 Matrix/4
  Constant2/1 -> Create 3x3 Matrix/5
  Constant3/1 -> Create 3x3 Matrix/6
  Trigonometric Function2/1 -> Create 3x3 Matrix/3, Unary Minus/1
  Unary Minus/1 -> Create 3x3 Matrix/7
  Constant4/1 -> Create 3x3 Matrix/8
  Trigonometric Function2/2 -> Create 3x3 Matrix/1, Create 3x3 Matrix/9
  alpha/1 -> Trigonometric Function2/1

== system DatcomNew/My Digital DATCOM v1.0.1/Dynamic Contribution/Aerodynamic Forces and Moments Stability Axis/Force Transformation/Incidence, Sideslip, & Airspeed ==
  Vb : Inport  Unit=m/s
  Airspeed : Sqrt  AlgorithmType=Newton-Raphson  SaturateOnIntegerOverflow=on
  Dot Product : DotProduct  InputSameDT=on  OutDataTypeStr=Inherit: Inherit via internal rule
  Incidence : Trigonometry  Operator=atan2
  Product : Product  Inputs=*/  SaturateOnIntegerOverflow=on  OutDataTypeStr=Inherit: Same as first input
  Selector : Selector  InputPortWidth=3  IndexOptions=Index vector (dialog)  Indices=[2]  OutputSizes=1
  Selector1 : Selector  InputPortWidth=3  IndexOptions=Index vector (dialog)  Indices=[3]  OutputSizes=1
  Selector2 : Selector  InputPortWidth=3  IndexOptions=Index vector (dialog)  Indices=[1]  OutputSizes=1
  Sideslip : Trigonometry  Operator=asin
  Alpha : Outport  Unit=rad  InitialOutput=0
  Beta : Outport  Port=2  Unit=rad  InitialOutput=0
  V : Outport  Port=3  Unit=m/s  InitialOutput=0
  wires:
  Product/1 -> Sideslip/1
  Selector1/1 -> Incidence/1
  Selector2/1 -> Incidence/2
  Dot Product/1 -> Airspeed/1
  Airspeed/1 -> Product/2, V/1
  Incidence/1 -> Alpha/1
  Vb/1 -> Selector1/1, Selector2/1, Selector/1, Dot Product/1, Dot Product/2
  Sideslip/1 -> Beta/1
  Selector/1 -> Product/1

== system DatcomNew/My Digital DATCOM v1.0.1/Dynamic Contribution/Aerodynamic Forces and Moments Stability Axis/Moment Transformation/Body2Stability ==
  alpha : Inport
  Constant{,1,3..4} (4 alike) : Constant  Value=0
  Constant2 : Constant
  Create 3x3 Matrix : aerolibutil/Create 3x3 Matrix
      settings: SourceProductName=Aerospace Blockset  SourceProductBaseCode=AE
  Trigonometric Function2 : Trigonometry  Operator=sincos
  Unary Minus : UnaryMinus
  Ts/b : Outport
  wires:
  alpha/1 -> Trigonometric Function2/1
  Trigonometric Function2/2 -> Create 3x3 Matrix/9, Create 3x3 Matrix/1
  Constant4/1 -> Create 3x3 Matrix/8
  Unary Minus/1 -> Create 3x3 Matrix/7
  Trigonometric Function2/1 -> Unary Minus/1, Create 3x3 Matrix/3
  Constant3/1 -> Create 3x3 Matrix/6
  Constant2/1 -> Create 3x3 Matrix/5
  Constant1/1 -> Create 3x3 Matrix/4
  Constant/1 -> Create 3x3 Matrix/2
  Create 3x3 Matrix/1 -> Ts/b/1

== system DatcomNew/My Digital DATCOM v1.0.1/Dynamic Contribution/Aerodynamic Forces and Moments Stability Axis/Moment Transformation/Incidence, Sideslip, & Airspeed ==
  Vb : Inport  Unit=m/s
  Airspeed : Sqrt  AlgorithmType=Newton-Raphson  SaturateOnIntegerOverflow=on
  Dot Product : DotProduct  InputSameDT=on  OutDataTypeStr=Inherit: Inherit via internal rule
  Incidence : Trigonometry  Operator=atan2
  Product : Product  Inputs=*/  SaturateOnIntegerOverflow=on  OutDataTypeStr=Inherit: Same as first input
  Selector : Selector  InputPortWidth=3  IndexOptions=Index vector (dialog)  Indices=[2]  OutputSizes=1
  Selector1 : Selector  InputPortWidth=3  IndexOptions=Index vector (dialog)  Indices=[3]  OutputSizes=1
  Selector2 : Selector  InputPortWidth=3  IndexOptions=Index vector (dialog)  Indices=[1]  OutputSizes=1
  Sideslip : Trigonometry  Operator=asin
  Alpha : Outport  Unit=rad  InitialOutput=0
  Beta : Outport  Port=2  Unit=rad  InitialOutput=0
  V : Outport  Port=3  Unit=m/s  InitialOutput=0
  wires:
  Selector/1 -> Product/1
  Sideslip/1 -> Beta/1
  Vb/1 -> Dot Product/2, Dot Product/1, Selector/1, Selector2/1, Selector1/1
  Incidence/1 -> Alpha/1
  Airspeed/1 -> V/1, Product/2
  Dot Product/1 -> Airspeed/1
  Selector2/1 -> Incidence/2
  Selector1/1 -> Incidence/1
  Product/1 -> Sideslip/1

== system DatcomNew/My Digital DATCOM v1.0.1/Static Contribution/Aerodynamic Forces and Moments/CG-CP Transformation/Body2Stability ==
  alpha : Inport
  Constant{,1,3..4} (4 alike) : Constant  Value=0
  Constant2 : Constant
  Create 3x3 Matrix : aerolibutil/Create 3x3 Matrix
      settings: SourceProductName=Aerospace Blockset  SourceProductBaseCode=AE
  Trigonometric Function2 : Trigonometry  Operator=sincos
  Unary Minus : UnaryMinus
  Ts/b : Outport
  wires:
  Create 3x3 Matrix/1 -> Ts/b/1
  Constant/1 -> Create 3x3 Matrix/2
  Constant1/1 -> Create 3x3 Matrix/4
  Constant2/1 -> Create 3x3 Matrix/5
  Constant3/1 -> Create 3x3 Matrix/6
  Trigonometric Function2/1 -> Create 3x3 Matrix/3, Unary Minus/1
  Unary Minus/1 -> Create 3x3 Matrix/7
  Constant4/1 -> Create 3x3 Matrix/8
  Trigonometric Function2/2 -> Create 3x3 Matrix/1, Create 3x3 Matrix/9
  alpha/1 -> Trigonometric Function2/1

== system DatcomNew/My Digital DATCOM v1.0.1/Static Contribution/Aerodynamic Forces and Moments/CG-CP Transformation/Incidence, Sideslip, & Airspeed ==
  Vb : Inport  Unit=m/s
  Airspeed : Sqrt  AlgorithmType=Newton-Raphson  SaturateOnIntegerOverflow=on
  Dot Product : DotProduct  InputSameDT=on  OutDataTypeStr=Inherit: Inherit via internal rule
  Incidence : Trigonometry  Operator=atan2
  Product : Product  Inputs=*/  SaturateOnIntegerOverflow=on  OutDataTypeStr=Inherit: Same as first input
  Selector : Selector  InputPortWidth=3  IndexOptions=Index vector (dialog)  Indices=[2]  OutputSizes=1
  Selector1 : Selector  InputPortWidth=3  IndexOptions=Index vector (dialog)  Indices=[3]  OutputSizes=1
  Selector2 : Selector  InputPortWidth=3  IndexOptions=Index vector (dialog)  Indices=[1]  OutputSizes=1
  Sideslip : Trigonometry  Operator=asin
  Alpha : Outport  Unit=rad  InitialOutput=0
  Beta : Outport  Port=2  Unit=rad  InitialOutput=0
  V : Outport  Port=3  Unit=m/s  InitialOutput=0
  wires:
  Product/1 -> Sideslip/1
  Selector1/1 -> Incidence/1
  Selector2/1 -> Incidence/2
  Dot Product/1 -> Airspeed/1
  Airspeed/1 -> Product/2, V/1
  Incidence/1 -> Alpha/1
  Vb/1 -> Selector1/1, Selector2/1, Selector/1, Dot Product/1, Dot Product/2
  Sideslip/1 -> Beta/1
  Selector/1 -> Product/1

== system DatcomNew/My Digital DATCOM v1.0.1/Static Contribution/Aerodynamic Forces and Moments/Force Transformation/Body2Stability ==
  alpha : Inport
  Constant{,1,3..4} (4 alike) : Constant  Value=0
  Constant2 : Constant
  Create 3x3 Matrix : aerolibutil/Create 3x3 Matrix
      settings: SourceProductName=Aerospace Blockset  SourceProductBaseCode=AE
  Trigonometric Function2 : Trigonometry  Operator=sincos
  Unary Minus : UnaryMinus
  Ts/b : Outport
  wires:
  Create 3x3 Matrix/1 -> Ts/b/1
  Constant/1 -> Create 3x3 Matrix/2
  Constant1/1 -> Create 3x3 Matrix/4
  Constant2/1 -> Create 3x3 Matrix/5
  Constant3/1 -> Create 3x3 Matrix/6
  Trigonometric Function2/1 -> Create 3x3 Matrix/3, Unary Minus/1
  Unary Minus/1 -> Create 3x3 Matrix/7
  Constant4/1 -> Create 3x3 Matrix/8
  Trigonometric Function2/2 -> Create 3x3 Matrix/1, Create 3x3 Matrix/9
  alpha/1 -> Trigonometric Function2/1

== system DatcomNew/My Digital DATCOM v1.0.1/Static Contribution/Aerodynamic Forces and Moments/Force Transformation/Incidence, Sideslip, & Airspeed ==
  Vb : Inport  Unit=m/s
  Airspeed : Sqrt  AlgorithmType=Newton-Raphson  SaturateOnIntegerOverflow=on
  Dot Product : DotProduct  InputSameDT=on  OutDataTypeStr=Inherit: Inherit via internal rule
  Incidence : Trigonometry  Operator=atan2
  Product : Product  Inputs=*/  SaturateOnIntegerOverflow=on  OutDataTypeStr=Inherit: Same as first input
  Selector : Selector  InputPortWidth=3  IndexOptions=Index vector (dialog)  Indices=[2]  OutputSizes=1
  Selector1 : Selector  InputPortWidth=3  IndexOptions=Index vector (dialog)  Indices=[3]  OutputSizes=1
  Selector2 : Selector  InputPortWidth=3  IndexOptions=Index vector (dialog)  Indices=[1]  OutputSizes=1
  Sideslip : Trigonometry  Operator=asin
  Alpha : Outport  Unit=rad  InitialOutput=0
  Beta : Outport  Port=2  Unit=rad  InitialOutput=0
  V : Outport  Port=3  Unit=m/s  InitialOutput=0
  wires:
  Product/1 -> Sideslip/1
  Selector1/1 -> Incidence/1
  Selector2/1 -> Incidence/2
  Dot Product/1 -> Airspeed/1
  Airspeed/1 -> Product/2, V/1
  Incidence/1 -> Alpha/1
  Vb/1 -> Selector1/1, Selector2/1, Selector/1, Dot Product/1, Dot Product/2
  Sideslip/1 -> Beta/1
  Selector/1 -> Product/1

== system DatcomNew/My Digital DATCOM v1.0.1/Static Contribution/Aerodynamic Forces and Moments/Moment Transformation/Body2Stability ==
  alpha : Inport
  Constant{,1,3..4} (4 alike) : Constant  Value=0
  Constant2 : Constant
  Create 3x3 Matrix : aerolibutil/Create 3x3 Matrix
      settings: SourceProductName=Aerospace Blockset  SourceProductBaseCode=AE
  Trigonometric Function2 : Trigonometry  Operator=sincos
  Unary Minus : UnaryMinus
  Ts/b : Outport
  wires:
  alpha/1 -> Trigonometric Function2/1
  Trigonometric Function2/2 -> Create 3x3 Matrix/9, Create 3x3 Matrix/1
  Constant4/1 -> Create 3x3 Matrix/8
  Unary Minus/1 -> Create 3x3 Matrix/7
  Trigonometric Function2/1 -> Unary Minus/1, Create 3x3 Matrix/3
  Constant3/1 -> Create 3x3 Matrix/6
  Constant2/1 -> Create 3x3 Matrix/5
  Constant1/1 -> Create 3x3 Matrix/4
  Constant/1 -> Create 3x3 Matrix/2
  Create 3x3 Matrix/1 -> Ts/b/1
